simulink model "Guia01"  (R2017b)
settings: Solver=VariableStepAuto  StartTime=0.0  StopTime=20.0  RelTol=1e-3
settings Model: Creator=Manu  LastModifiedBy=Manu

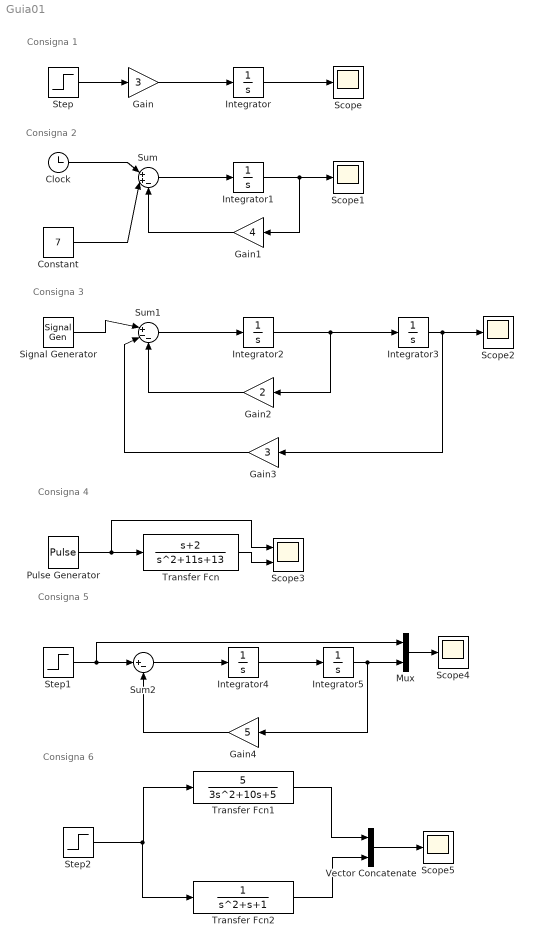
== system Guia01 ==
  note: Consigna 3
  note: Consigna 2
  note: Consigna 1
  note: Consigna 4
  note: Consigna 5
  note: Consigna 6
  Clock : Clock
  Constant : Constant  Value=7
  Gain : Gain  Gain=3
  Gain1 : Gain  Gain=4
  Gain2 : Gain  Gain=2
  Gain3 : Gain  Gain=3
  Gain4 : Gain  Gain=5
  Integrator{,1..5} (6 alike) : Integrator
  Mux : Mux  Inputs=2
  Pulse Generator : DiscretePulseGenerator  PulseType=Time based  Amplitude=3  Period=10  PulseWidth=50
  Scope{,1..2,4..5} (5 alike) : Scope
  Scope3 : Scope  NumInputPorts=2
  Signal Generator : SignalGenerator  Frequency=500  Units=rad/sec
  Step : Step  Time=2  SampleTime=0
  Step1 : Step  SampleTime=0
  Step2 : Step  SampleTime=0
  Sum : Sum  Inputs=|++-
  Sum1 : Sum  Inputs=|+--
  Sum2 : Sum  Inputs=|+-
  Transfer Fcn : TransferFcn  Numerator=[1 2]  Denominator=[1 11 13]
  Transfer Fcn1 : TransferFcn  Numerator=[5]  Denominator=[3 10 5]
  Transfer Fcn2 : TransferFcn  Denominator=[1 1 1]
  Vector Concatenate : Concatenate
  wires:
  Step/1 -> Gain/1
  Gain/1 -> Integrator/1
  Clock/1 -> Sum/1
  Constant/1 -> Sum/2
  Gain1/1 -> Sum/3
  Integrator1/1 -> Gain1/1, Scope1/1
  Sum/1 -> Integrator1/1
  Integrator/1 -> Scope/1
  Signal Generator/1 -> Sum1/1
  Gain3/1 -> Sum1/2
  Gain2/1 -> Sum1/3
  Sum1/1 -> Integrator2/1
  Integrator2/1 -> Gain2/1, Integrator3/1
  Integrator3/1 -> Scope2/1, Gain3/1
  Transfer Fcn/1 -> Scope3/2
  Pulse Generator/1 -> Transfer Fcn/1, Scope3/1
  Sum2/1 -> Integrator4/1
  Integrator4/1 -> Integrator5/1
  Integrator5/1 -> Mux/2, Gain4/1
  Gain4/1 -> Sum2/2
  Step1/1 -> Mux/1, Sum2/1
  Mux/1 -> Scope4/1
  Step2/1 -> Transfer Fcn2/1, Transfer Fcn1/1
  Transfer Fcn1/1 -> Vector Concatenate/1
  Transfer Fcn2/1 -> Vector Concatenate/2
  Vector Concatenate/1 -> Scope5/1
